simulink model "controlModel"  (R2015a)
settings: Solver=ode45  StartTime=0.0  StopTime=50  RelTol=1e-3
values from neighbouring files (symbols this model uses):
  Ch = 9    [script.m]
  Ke = -1.0000e+05    (= -100000)    [script.m]
  Kh = 625    [script.m]
  L = motor*cart    [script.m]
  M = 1.35    [script.m]
  R = 1.3    [script.m]
undefined symbols (not defined in the file or in its folder): i
settings Model: Creator=jinkale  LastModifiedBy=jinkale

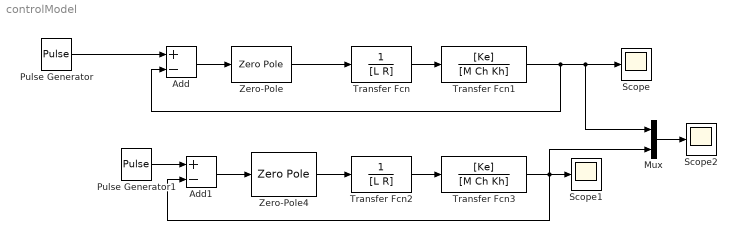
== system controlModel ==
  Add : Sum  Inputs=+-
  Add1 : Sum  Inputs=+-
  Mux : Mux  Inputs=2
  Pulse Generator : DiscretePulseGenerator  PulseType=Time based  Amplitude=3  Period=10  PulseWidth=50
  Pulse Generator1 : DiscretePulseGenerator  PulseType=Time based  Amplitude=3  Period=10  PulseWidth=50
  Scope : Scope
      settings: TimeRange=50  YMin=-1  YMax=4  MaxDataPoints=500000
  Scope1 : Scope
      settings: TimeRange=50  YMin=-1  YMax=4  MaxDataPoints=500000
  Scope2 : Scope
      settings: TimeRange=50  YMin=-1  YMax=4  SaveName=ScopeData2  MaxDataPoints=500000
  Transfer Fcn : TransferFcn  Denominator=[L R]
  Transfer Fcn1 : TransferFcn  Numerator=[Ke]  Denominator=[M Ch Kh]
  Transfer Fcn2 : TransferFcn  Denominator=[L R]
  Transfer Fcn3 : TransferFcn  Numerator=[Ke]  Denominator=[M Ch Kh]
  Zero-Pole : ZeroPole  Zeros=[3.0405+i*12.6,3.0405-i*12.6]  Poles=[0 -200]  Gain=[-0.038702*560]
  Zero-Pole4 : ZeroPole  Zeros=[9.52+3.16i,9.52-3.16i]  Poles=[0,-100]  Gain=-0.016498*560
  wires:
  Pulse Generator/1 -> Add/1
  Transfer Fcn1/1 -> Add/2, Mux/1, Scope/1
  Transfer Fcn/1 -> Transfer Fcn1/1
  Add/1 -> Zero-Pole/1
  Zero-Pole/1 -> Transfer Fcn/1
  Add1/1 -> Zero-Pole4/1
  Zero-Pole4/1 -> Transfer Fcn2/1
  Transfer Fcn2/1 -> Transfer Fcn3/1
  Pulse Generator1/1 -> Add1/1
  Transfer Fcn3/1 -> Mux/2, Add1/2, Scope1/1
  Mux/1 -> Scope2/1
